simulink model "Simulink_Imlemented_2DKF_Plane_tracking"  (R2022b)
settings: Solver=FixedStepDiscrete  StartTime=0.0  StopTime=4  FixedStep=dt  RelTol=1e-3
undefined symbols (not defined in the file): a, A, B, C, Discrete, dt, H, P0, R, Time, yM
libraries: ctrlSharedLib x1
settings Model: Creator=leoni  LastModifiedBy=leoni

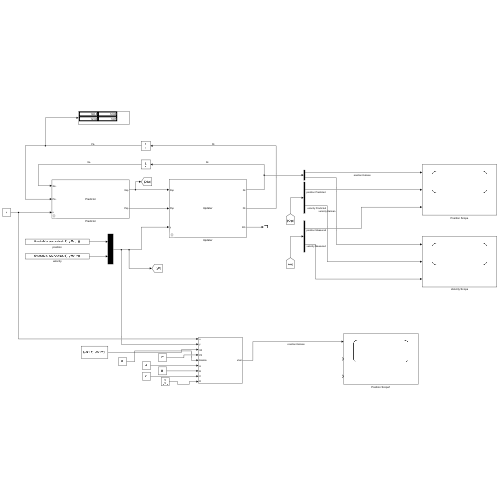
[thumbnail: Simulink's stored preview of the top-level diagram]
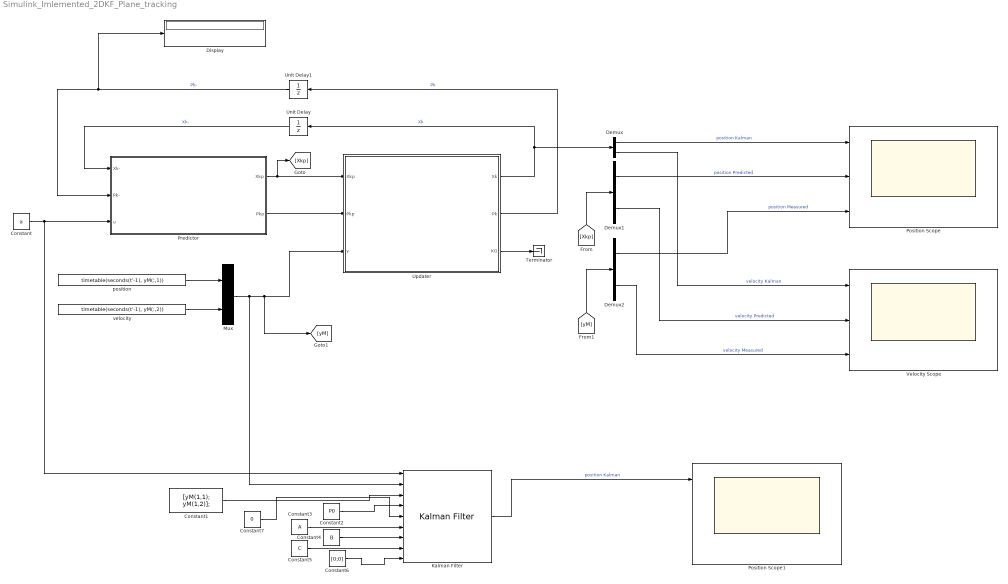
== system Simulink_Imlemented_2DKF_Plane_tracking ==
  Constant : Constant  Value=a
  Constant1 : Constant  Value=[yM(1,1); yM(1,2)];  VectorParams1D=off  SampleTime=-1
  Constant2 : Constant  Value=P0  VectorParams1D=off
  Constant3 : Constant  Value=A  VectorParams1D=off
  Constant4 : Constant  Value=B  VectorParams1D=off
  Constant5 : Constant  Value=C  VectorParams1D=off
  Constant6 : Constant  Value=[0;0]  VectorParams1D=off
  Constant7 : Constant  Value=0
  Demux : Demux  Outputs=2
  Demux1 : Demux  Outputs=2
  Demux2 : Demux  Outputs=2
  Display : Display
  Kalman Filter : ctrlSharedLib/Kalman Filter  TimeDomain=Discrete-Time  UseCurrentEstimator=on  ModelSource=Input port  ModelSourceVariable=ss(0.95,1,1,0,1)  A=A  B=B  C=C  D=0  NumberOfStates=2  NumberOfInputs=1  NumberOfOutputs=2  InitialEstimateSource=Input port  X0=0  P0=10  UseK=off  UseGH=off  NumberOfProcessNoiseInputs=1  G=1  TimeInvariantG=on  H=0  TimeInvariantH=on  Q=0  TimeInvariantQ=on  R=R  TimeInvariantR=on  N=0  TimeInvariantN=on  AddInputPort=on  AddEnablePort=on  OutputEstimatedY=off  OutputP=off  Ts=-1
  Mux : Mux  Inputs=2
  Position Scope : Scope  NumInputPorts=3
  Position Scope1 : Scope  NumInputPorts=3
  Predictor : Subsystem
      mask Display: disp('Predictor')
  Terminator : Terminator
  Unit Delay : UnitDelay  InitialCondition=[yM(1,1); yM(1,2)];  SampleTime=-1  HasFrameUpgradeWarning=on
  Unit Delay1 : UnitDelay  InitialCondition=P0  SampleTime=-1  HasFrameUpgradeWarning=on
  Updater : Subsystem
      mask Display: disp('Updater')
  Velocity Scope : Scope  NumInputPorts=3
  position : FromWorkspace  VariableName=timetable(seconds(t'-1), yM(:,1))  SampleTime=1  Interpolate=off  OutputAfterFinalValue=Holding final value
  velocity : FromWorkspace  VariableName=timetable(seconds(t'-1), yM(:,2))  SampleTime=1  Interpolate=off  OutputAfterFinalValue=Holding final value
  wires:
  Predictor/1(Xkp) -> Updater/1(Xkp), [Xkp]
  Predictor/2(Pkp) -> Updater/2(Pkp)
  Updater/1(Xk) -> Demux/1, Unit Delay/1  "Xk"
  Updater/2(Pk) -> Unit Delay1/1  "Pk"
  Unit Delay/1 -> Predictor/1(Xk-)  "Xk-"
  Unit Delay1/1 -> Display/1, Predictor/2(Pk-)  "Pk-"
  Updater/3(KG) -> Terminator/1
  velocity/1 -> Mux/2
  Mux/1 -> Kalman Filter/2, [yM], Updater/3(y)
  Demux/1 -> Position Scope/1  "position Kalman"
  Demux/2 -> Velocity Scope/1  "velocity Kalman"
  [Xkp] -> Demux1/1
  Demux1/1 -> Position Scope/2  "position Predicted"
  Demux1/2 -> Velocity Scope/2  "velocity Predicted"
  position/1 -> Mux/1
  [yM] -> Demux2/1
  Demux2/1 -> Position Scope/3  "position Measured"
  Demux2/2 -> Velocity Scope/3  "velocity Measured"
  Kalman Filter/1 -> Position Scope1/1  "position Kalman"
  Constant1/1 -> Kalman Filter/3
  Constant2/1 -> Kalman Filter/4
  Constant3/1 -> Kalman Filter/6
  Constant4/1 -> Kalman Filter/7
  Constant5/1 -> Kalman Filter/8
  Constant6/1 -> Kalman Filter/9
  Constant/1 -> Kalman Filter/1, Predictor/3(u)
  Constant7/1 -> Kalman Filter/5

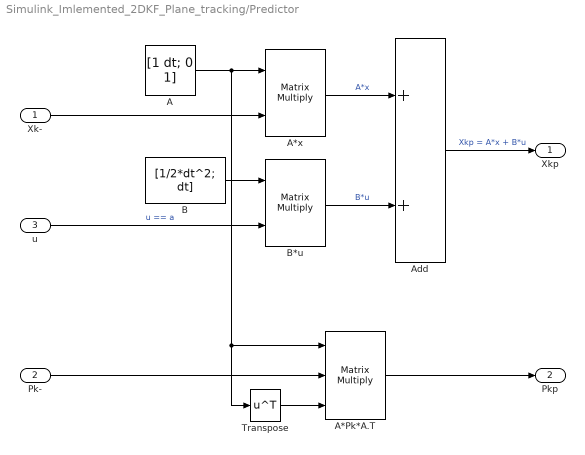
== system Simulink_Imlemented_2DKF_Plane_tracking/Predictor ==
  Xk- : Inport
  Pk- : Inport  Port=2
  u : Inport  Port=3
  A : Constant  Value=[1 dt; 0 1]  VectorParams1D=off
  A*Pk*A.T : Product  Inputs=***  Multiplication=Matrix(*)
  A*x : Product  Inputs=**  Multiplication=Matrix(*)
  Add : Sum
  B : Constant  Value=[1/2*dt^2; dt]  VectorParams1D=off
  B*u : Product  Inputs=**  Multiplication=Matrix(*)
  Transpose : Math  Operator=transpose
  Xkp : Outport
  Pkp : Outport  Port=2
  wires:
  Xk-/1 -> A*x/2
  A/1 -> Transpose/1, A*Pk*A.T/1, A*x/1
  u/1 -> B*u/2  "u == a"
  B/1 -> B*u/1
  A*x/1 -> Add/1  "A*x"
  B*u/1 -> Add/2  "B*u"
  Add/1 -> Xkp/1  "Xkp = A*x + B*u"
  Pk-/1 -> A*Pk*A.T/2
  Transpose/1 -> A*Pk*A.T/3
  A*Pk*A.T/1 -> Pkp/1

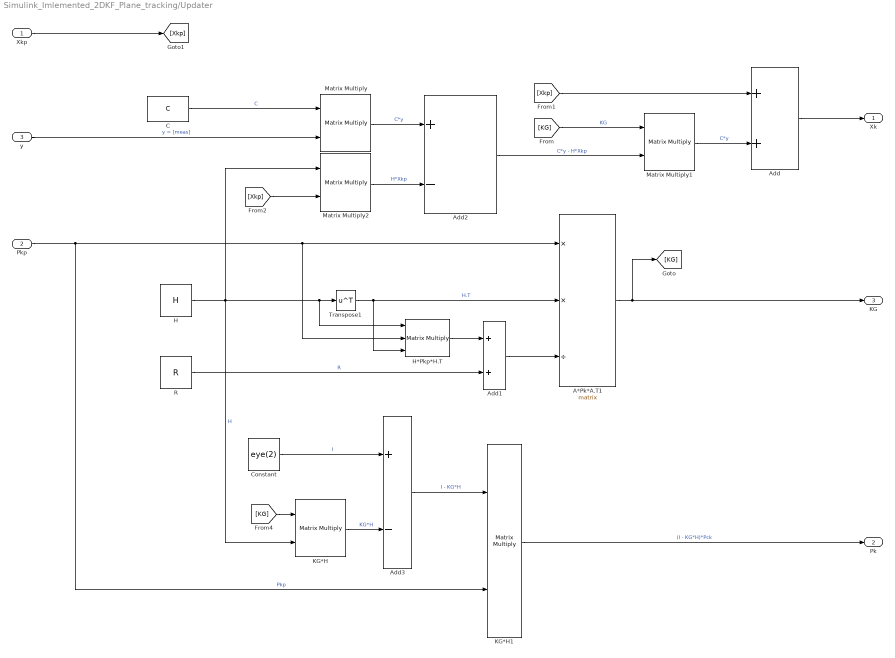
== system Simulink_Imlemented_2DKF_Plane_tracking/Updater ==
  Xkp : Inport
  Pkp : Inport  Port=2
  y : Inport  Port=3
  A*Pk*A.T1 : Product  Inputs=**/  Multiplication=Matrix(*)
  Add : Sum
  Add1 : Sum
  Add2 : Sum  Inputs=+-
  Add3 : Sum  Inputs=+-
  C : Constant  Value=C  VectorParams1D=off
  Constant : Constant  Value=eye(2)
  H : Constant  Value=H  VectorParams1D=off
  H*Pkp*H.T : Product  Inputs=***  Multiplication=Matrix(*)
  KG*H : Product  Multiplication=Matrix(*)
  KG*H1 : Product  Multiplication=Matrix(*)
  Matrix Multiply : Product  Multiplication=Matrix(*)
  Matrix Multiply1 : Product  Multiplication=Matrix(*)
  Matrix Multiply2 : Product  Multiplication=Matrix(*)
  R : Constant  Value=R  VectorParams1D=off
  Transpose1 : Math  Operator=transpose
  Xk : Outport
  Pk : Outport  Port=2
  KG : Outport  Port=3
  wires:
  Pkp/1 -> KG*H1/2, H*Pkp*H.T/2, A*Pk*A.T1/1  "Pkp"
  Transpose1/1 -> H*Pkp*H.T/3, A*Pk*A.T1/2  "H.T"
  H/1 -> KG*H/2, Matrix Multiply2/1, Transpose1/1, H*Pkp*H.T/1  "H"
  H*Pkp*H.T/1 -> Add1/1
  R/1 -> Add1/2  "R"
  Add1/1 -> A*Pk*A.T1/3
  A*Pk*A.T1/1 -> [KG], KG/1
  Xkp/1 -> [Xkp]
  y/1 -> Matrix Multiply/2  "y = [meas]"
  C/1 -> Matrix Multiply/1  "C"
  Matrix Multiply/1 -> Add2/1  "C*y"
  Matrix Multiply2/1 -> Add2/2  "H*Xkp"
  Add2/1 -> Matrix Multiply1/2  "C*y - H*Xkp"
  [Xkp] -> Add/1
  [KG] -> Matrix Multiply1/1  "KG"
  Matrix Multiply1/1 -> Add/2  "C*y"
  Add/1 -> Xk/1
  [Xkp] -> Matrix Multiply2/2
  Constant/1 -> Add3/1  "I"
  Add3/1 -> KG*H1/1  "I - KG*H"
  [KG] -> KG*H/1
  KG*H/1 -> Add3/2  "KG*H"
  KG*H1/1 -> Pk/1  "(I - KG*H)*Pck"
